simulink model "Modelo_Primer_orden_Obtencion_datos"  (R2016a)
settings: Solver=VariableStepAuto  StartTime=0.0  StopTime=10.0  RelTol=1e-3
settings Model: Creator=Daniel  LastModifiedBy=Daniel

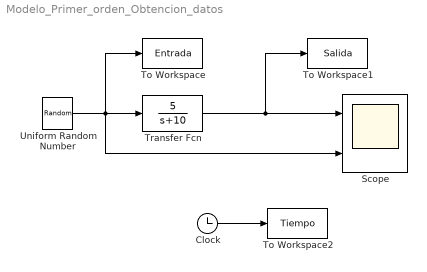
== system Modelo_Primer_orden_Obtencion_datos ==
  Clock : Clock
  Scope : Scope  NumInputPorts=2
  To Workspace : ToWorkspace  VariableName=Entrada  SampleTime=0.01
  To Workspace1 : ToWorkspace  VariableName=Salida  SampleTime=0.01
  To Workspace2 : ToWorkspace  VariableName=Tiempo  SampleTime=0.01
  Transfer Fcn : TransferFcn  Numerator=[5]  Denominator=[1 10]
  Uniform Random Number : UniformRandomNumber  Minimum=0  Maximum=5  SampleTime=0.5
  wires:
  Uniform Random Number/1 -> Scope/2, To Workspace/1, Transfer Fcn/1
  Transfer Fcn/1 -> To Workspace1/1, Scope/1
  Clock/1 -> To Workspace2/1
